simulink model "check_Clutch"  (R2018b)
settings: configuration reference "Physics" (kept outside this file)
model workspace (MAT data in the model file):
  veh_param = Simulink.Parameter
  veh_param.Value.cLiftF = 0
  veh_param.Value.cLiftR = 0
  veh_param.Value.CoGx_m = 0
  veh_param.Value.CoGy_m = 0
  veh_param.Value.CoGz_m = 0
  veh_param.Value.cDrag = 0
  veh_param.Value.Aref_m2 = 0
  veh_param.Value.Gearratio = 0
  veh_param.Value.Wheelbase_m = 0
  veh_param.Value.PacLatF = [0 0 0 0 0]
  veh_param.Value.PacLongF = [0 0 0 0 0]
  veh_param.Value.PacLatR = [0 0 0 0 0]
  veh_param.Value.PacLongR = [0 0 0 0 0]
  veh_param.Value.cRollFriction_Npmps = 0
  veh_param.Value.MaxRollFriction_N = 0
  veh_param.Value.T_YawRate_s = 0
  veh_param.Value.T_LatVel_s = 0
  veh_param.Value.TrackWidthF_m = 0
  veh_param.Value.TrackWidthR_m = 0
  veh_param.Value.TireRadiusF_m = 0
  veh_param.Value.TireRadiusR_m = 0
  veh_param.Value.VehicleInertia_kgm2 = 0
  veh_param.Value.WheelInertiaF_kgm2 = 0
  veh_param.Value.WheelInertiaR_kgm2 = 0
  veh_param.Value.VehicleMass_kg = 0
  veh_param.Value.switchModelBlend_mps = 0
  veh_param.Value.PTLimitLowVel_N = 0
  veh_param.Value.switchModelVel_mps = 0
  veh_param.Value.T_Tire_s = 0
  veh_param.DataType = 'struct'
  veh_param.Dimensions = [1 1]
  x0_positionstates = Simulink.Parameter
  x0_positionstates.Value = [0 0 0]
  x0_positionstates.DataType = 'auto'
  x0_positionstates.Dimensions = [1 3]
undefined symbols (not defined in the file): POWTR__CLUTCH__clutch_time_s, POWTR__CLUTCH__T_max_cap_Nm, POWTR__DIFFERENTIAL__I_drivetrain_kgm2, POWTR__ENGINE__I_engine_kgm2, POWTR__ENGINE__n_0_rpm, POWTR__TRANSMISSION__I_transmission_kgm2
settings Model: DataDictionary=vehicleparameters_vehdynsim.sldd  OrderedModelArguments=off  Creator=wischnewski  LastModifiedBy=ga25xiw

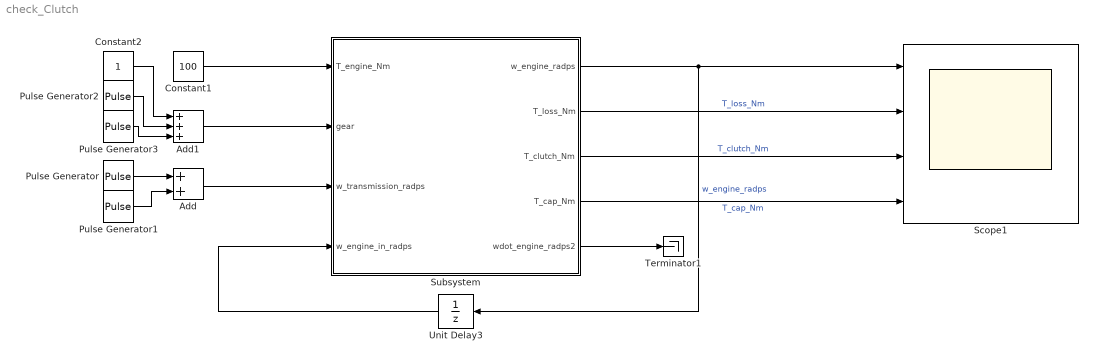
== system check_Clutch ==
  Add : Sum
  Add1 : Sum  Inputs=+++
  Constant1 : Constant  Value=100
  Constant2 : Constant
  Pulse Generator : DiscretePulseGenerator  PulseType=Time based  Amplitude=400  Period=10  PulseWidth=90  PhaseDelay=3
  Pulse Generator1 : DiscretePulseGenerator  PulseType=Time based  Amplitude=-200  Period=10  PulseWidth=90  PhaseDelay=6
  Pulse Generator2 : DiscretePulseGenerator  PulseType=Time based  Period=10  PulseWidth=90  PhaseDelay=3
  Pulse Generator3 : DiscretePulseGenerator  PulseType=Time based  Amplitude=-1  Period=10  PulseWidth=90  PhaseDelay=6
  Scope1 : Scope  NumInputPorts=4
  Subsystem : Subsystem
  Terminator1 : Terminator
  Unit Delay3 : UnitDelay  SampleTime=-1
  wires:
  Unit Delay3/1 -> Subsystem/4(w_engine_in_radps)
  Subsystem/1(w_engine_radps) -> Scope1/1, Unit Delay3/1  "w_engine_radps"
  Subsystem/2(T_loss_Nm) -> Scope1/2  "T_loss_Nm"
  Subsystem/3(T_clutch_Nm) -> Scope1/3  "T_clutch_Nm"
  Add/1 -> Subsystem/3(w_transmission_radps)
  Constant1/1 -> Subsystem/1(T_engine_Nm)
  Subsystem/4(T_cap_Nm) -> Scope1/4  "T_cap_Nm"
  Subsystem/5(wdot_engine_radps2) -> Terminator1/1
  Pulse Generator/1 -> Add/1
  Pulse Generator1/1 -> Add/2
  Add1/1 -> Subsystem/2(gear)
  Constant2/1 -> Add1/1
  Pulse Generator2/1 -> Add1/2
  Pulse Generator3/1 -> Add1/3

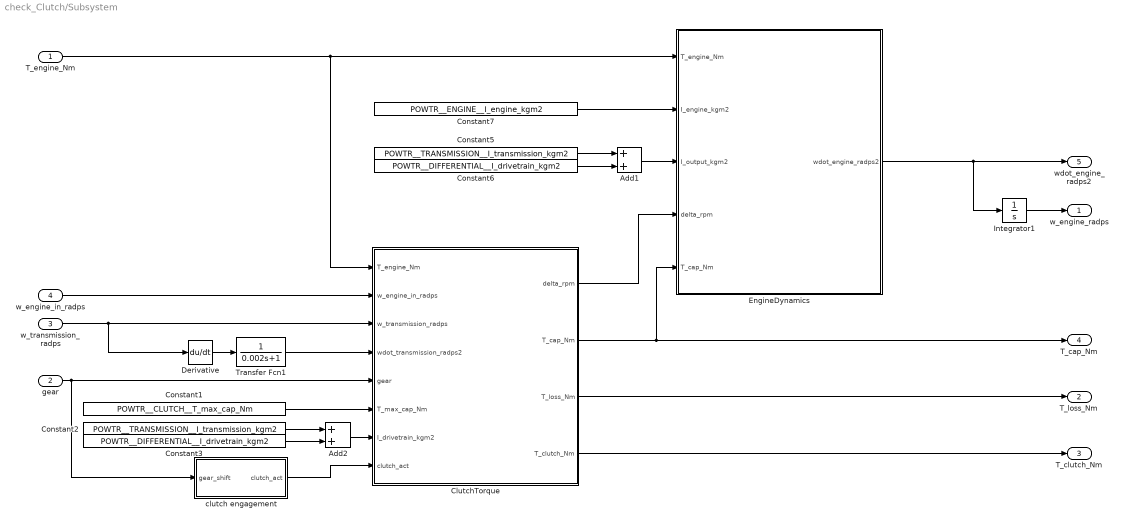
== system check_Clutch/Subsystem ==
  T_engine_Nm : Inport
  gear : Inport  Port=2
  w_transmission_radps : Inport  Port=3
  w_engine_in_radps : Inport  Port=4
  Add1 : Sum
  Add2 : Sum
  ClutchTorque : MATLAB Function  TreatAsAtomicUnit=on
  Constant1 : Constant  Value=POWTR__CLUTCH__T_max_cap_Nm
  Constant2 : Constant  Value=POWTR__TRANSMISSION__I_transmission_kgm2
  Constant3 : Constant  Value=POWTR__DIFFERENTIAL__I_drivetrain_kgm2
  Constant5 : Constant  Value=POWTR__TRANSMISSION__I_transmission_kgm2
  Constant6 : Constant  Value=POWTR__DIFFERENTIAL__I_drivetrain_kgm2
  Constant7 : Constant  Value=POWTR__ENGINE__I_engine_kgm2
  Derivative : Derivative
  EngineDynamics : MATLAB Function  TreatAsAtomicUnit=on
  Integrator1 : Integrator  InitialCondition=POWTR__ENGINE__n_0_rpm * ((2*pi)/60)
  Transfer Fcn1 : TransferFcn  Denominator=[0.002 1]
  clutch engagement : Subsystem
  w_engine_radps : Outport
  T_loss_Nm : Outport  Port=2
  T_clutch_Nm : Outport  Port=3
  T_cap_Nm : Outport  Port=4
  wdot_engine_radps2 : Outport  Port=5
  wires:
  Transfer Fcn1/1 -> ClutchTorque/4(wdot_transmission_radps2)
  Constant7/1 -> EngineDynamics/2(I_engine_kgm2)
  Constant5/1 -> Add1/1
  Constant6/1 -> Add1/2
  clutch engagement/1(clutch_act) -> ClutchTorque/8(clutch_act)
  ClutchTorque/1(delta_rpm) -> EngineDynamics/4(delta_rpm)
  ClutchTorque/3(T_loss_Nm) -> T_loss_Nm/1
  ClutchTorque/2(T_cap_Nm) -> T_cap_Nm/1, EngineDynamics/5(T_cap_Nm)
  ClutchTorque/4(T_clutch_Nm) -> T_clutch_Nm/1
  w_transmission_radps/1 -> Derivative/1, ClutchTorque/3(w_transmission_radps)
  Integrator1/1 -> w_engine_radps/1
  w_engine_in_radps/1 -> ClutchTorque/2(w_engine_in_radps)
  Constant1/1 -> ClutchTorque/6(T_max_cap_Nm)
  Derivative/1 -> Transfer Fcn1/1
  Add1/1 -> EngineDynamics/3(I_output_kgm2)
  gear/1 -> ClutchTorque/5(gear), clutch engagement/1(gear_shift)
  Add2/1 -> ClutchTorque/7(I_drivetrain_kgm2)
  T_engine_Nm/1 -> ClutchTorque/1(T_engine_Nm), EngineDynamics/1(T_engine_Nm)
  Constant2/1 -> Add2/1
  Constant3/1 -> Add2/2
  EngineDynamics/1(wdot_engine_radps2) -> Integrator1/1, wdot_engine_radps2/1

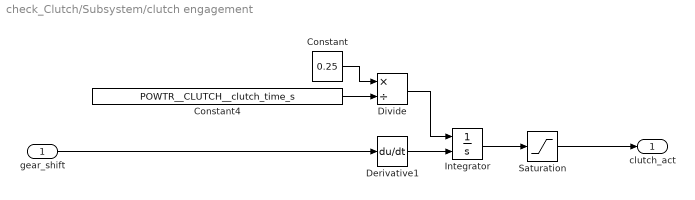
== system check_Clutch/Subsystem/clutch engagement ==
  gear_shift : Inport
  Constant : Constant  Value=0.25
  Constant4 : Constant  Value=POWTR__CLUTCH__clutch_time_s
  Derivative1 : Derivative
  Divide : Product  Inputs=*/
  Integrator : Integrator  ExternalReset=level hold
  Saturation : Saturate  UpperLimit=1  LowerLimit=0
  clutch_act : Outport
  wires:
  gear_shift/1 -> Derivative1/1
  Divide/1 -> Integrator/1
  Constant4/1 -> Divide/2
  Derivative1/1 -> Integrator/2
  Constant/1 -> Divide/1
  Integrator/1 -> Saturation/1
  Saturation/1 -> clutch_act/1

== matlab function check_Clutch/Subsystem/ClutchTorque ==
  data: T_engine_Nm input; delta_rpm output; w_engine_in_radps input; w_transmission_radps input; wdot_transmission_radps2 input; gear input; T_max_cap_Nm input; T_cap_Nm output; T_loss_Nm output; T_clutch_Nm output; I_drivetrain_kgm2 input; clutch_act input
function [delta_rpm, T_cap_Nm, T_loss_Nm, T_clutch_Nm] = fcn(T_engine_Nm, ...
                              w_engine_in_radps, w_transmission_radps, ...
                              wdot_transmission_radps2, gear, T_max_cap_Nm, ...
                              I_drivetrain_kgm2, clutch_act)

[delta_rpm, T_cap_Nm, T_loss_Nm, T_clutch_Nm] = ClutchTorque(T_engine_Nm, ...
                              w_engine_in_radps, w_transmission_radps, ...
                              wdot_transmission_radps2, gear, T_max_cap_Nm, ...
                              I_drivetrain_kgm2, clutch_act);

== matlab function check_Clutch/Subsystem/EngineDynamics ==
  data: T_engine_Nm input; I_engine_kgm2 input; I_output_kgm2 input; delta_rpm input; wdot_engine_radps2 output; T_cap_Nm input
function wdot_engine_radps2 = fcn(T_engine_Nm, I_engine_kgm2, ...
                              I_output_kgm2, delta_rpm, T_cap_Nm)

wdot_engine_radps2 = EngineDynamics(T_engine_Nm, I_engine_kgm2, ...
                              I_output_kgm2, delta_rpm, T_cap_Nm);
